simulink library "Grashof"  (Simulink 8.2)
settings: Solver=ode45  StartTime=0.0  StopTime=10.0  RelTol=1e-3
undefined symbols (not defined in the file): CarnotCallbacks_Grashof
settings Model: Creator=lena.frank  LastModifiedBy=drhf

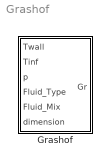
== system Grashof ==
  Grashof : Subsystem  LoadFcn=CarnotCallbacks_Grashof('LoadFcn');  VariantControl=CarlibClassic  mask(Grashof){DEBUGLEVEL=WARNINGLEVEL, MAXTOTALMESSAGES=inf, MAXCONSECUTIVEMESSAGES=inf, WRITETOFILE=0, FILENAME='errors.txt'}
      mask prompts: DEBUGLEVEL "Debug level"; MAXTOTALMESSAGES "maximum number of total warning"; MAXCONSECUTIVEMESSAGES "maximum number of consecutive warnings"; WRITETOFILE "write messages to file"; FILENAME "filename for error messages"
      mask help:
      | Calculates the Gashof number. You may use the block "GlobalMessageLevel" in the Toolbox to handle the debugging messages.
      | Inputs are:
      | 1   wall temperature - scalar or vector
      | 2   temperature at infinite distance - scalar
      | 3   pressure - scalar
      | 4   fluid type (see below) - scalar
      | 5   fluid_mix - scalar
      | 6   characteristic dimension - scalar
      |
      | FluidType        Remarks
      | 1: water          fluid mix is vapourcontent in the 2-phase region
      | 2: air              fluid mix is (kg water) / (kg dry air)
      | 3: cotton oil       -
      | 4: silicone oil     -
      | 5: water-glycol   fluid mix is volume partition [0..1] of propylen glycol
      | 6: Tyfocor LS     function only available in liquid phase
      | 7: Water Constant = 998.21 kg/m³ (water at 20°C)
      | 8: Air Constant   = 1.118 kg/m³ (air at 20°C)
      mask init:
      | %global debug level
      | [DEBUGLEVEL, MAXTOTALMESSAGES, MAXCONSECUTIVEMESSAGES, WRITETOFILE, FILENAME] = CarnotCallbacks_Grashof('CheckDebugLevels', DEBUGLEVEL, MAXTOTALMESSAGES, MAXCONSECUTIVEMESSAGES, WRITETOFILE, FILENAME);
      mask Help: web(fullfile(path_carnot('help'),'Grashof.html'),'-helpbrowser')
      mask TypeOptions DEBUGLEVEL: DEBUGLEVEL | INFOLEVEL | WARNINGLEVEL | ERRORLEVEL | FATALLEVEL | NOLEVEL
      mask DialogControl ParameterTabVar0 Prompt: Debugging

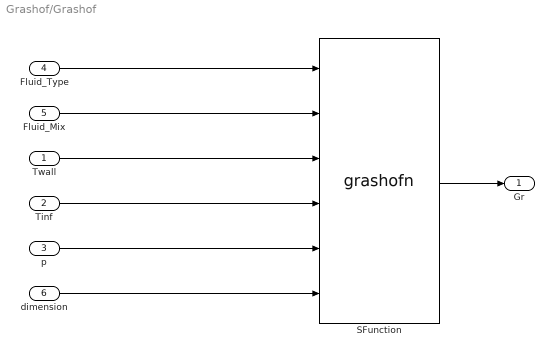
== system Grashof/Grashof ==
  Twall : Inport
  Tinf : Inport  Port=2
  p : Inport  Port=3
  Fluid_Type : Inport  Port=4
  Fluid_Mix : Inport  Port=5
  dimension : Inport  Port=6
  SFunction : S-Function  FunctionName=grashofn  Parameters=DEBUGLEVEL,MAXTOTALMESSAGES,MAXCONSECUTIVEMESSAGES,WRITETOFILE,FILENAME  EnableBusSupport=off
  Gr : Outport
  wires:
  dimension/1 -> SFunction/6
  p/1 -> SFunction/5
  Tinf/1 -> SFunction/4
  Twall/1 -> SFunction/3
  Fluid_Mix/1 -> SFunction/2
  Fluid_Type/1 -> SFunction/1
  SFunction/1 -> Gr/1
